simulink model "s3_22a"  (Simulink 6.6)
settings: Solver=FixedStepDiscrete  SolverMode=SingleTasking  StartTime=0.0  StopTime=t_d  FixedStep=Tc  MaxStep=Tc  RelTol=1e-6  AbsTol=1e-6
values from neighbouring files (symbols this model uses):
  a = [0.5; 0.5]    [i3_22.m]
  K = diag([500,500,500,100])    [i3_22.m]
  q_i = zeros(1,4)    [i3_22.m]
  Tc = 0.001    [i3_22.m]
  Ts = Tc    (= 0.001)    [i3_22.m]
undefined symbols (not defined in the file or in its folder): DiscIntNeverNeededParam
settings Model: Creator=luigivillani  LastModifiedBy=luigivillani  ExtModeAutoUpdateStatusClock=off
settings DataIOCC: LimitDataPoints=off  SaveOutput=off  SaveTime=off
settings OptimizationCC: BlockReduction=off  BooleanDataType=off
settings DebuggingCC: SignalResolutionControl=TryResolveAllWithWarning  SolverPrmCheckMsg=none  MultiTaskDSMMsg=warning  MultiTaskCondExecSysMsg=none  StrictBusMsg=None
settings HardwareCC: TargetUnknown=on
settings RTWCC: IncludeERTFirstTime=on

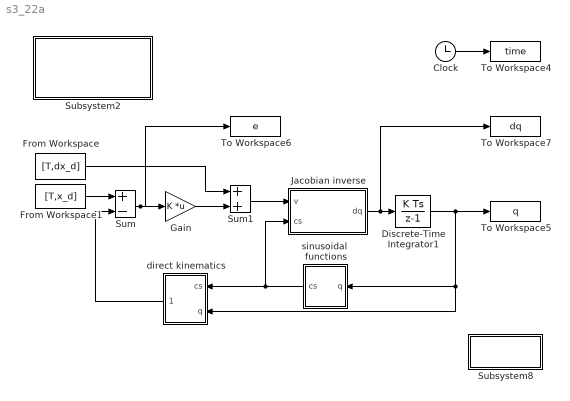
== system s3_22a ==
  Clock : Clock
  Discrete-Time Integrator1 : DiscreteIntegrator  InitialCondition=q_i  SampleTime=Tc  ICPrevOutput=DiscIntNeverNeededParam  ICPrevScaledInput=DiscIntNeverNeededParam
  From Workspace : FromWorkspace  VariableName=[T,dx_d]  SampleTime=Tc
  From Workspace1 : FromWorkspace  VariableName=[T,x_d]  SampleTime=Tc
  Gain : Gain  Gain=K  Multiplication=Matrix(K*u)  SampleTime=Tc
      mask Display: disp('K')
  Jacobian inverse : Subsystem
      mask Display: disp('inv(J_a(q))dx')
  Subsystem2 : Subsystem
      settings: OpenFcn=clear all;i3_22;
      mask Display: disp('variables\n initialization')
  Subsystem8 : Subsystem  Orientation=left
      settings: OpenFcn=p3_22a;
      mask Display: disp('plot')
  Sum : Sum  Inputs=+-  SaturateOnIntegerOverflow=on  InputSameDT=on
  Sum1 : Sum  SaturateOnIntegerOverflow=on  InputSameDT=on
  To Workspace4 : ToWorkspace  VariableName=time  SampleTime=Ts  SaveFormat=Array
      settings: MaxDataPoints=2501
  To Workspace5 : ToWorkspace  VariableName=q  SampleTime=Ts  SaveFormat=Array
      settings: MaxDataPoints=2501
  To Workspace6 : ToWorkspace  VariableName=e  SampleTime=Ts  SaveFormat=Array
      settings: MaxDataPoints=2501
  To Workspace7 : ToWorkspace  VariableName=dq  SampleTime=Ts  SaveFormat=Array
      settings: MaxDataPoints=2501
  direct kinematics : Subsystem  Orientation=left
      mask Display: disp('k(q)')
  sinusoidal  functions : Subsystem  Orientation=left
      mask Display: disp('cs(q)')
  wires:
  From Workspace1/1 -> Sum/1
  Clock/1 -> To Workspace4/1
  Gain/1 -> Sum1/2
  direct kinematics/1((x,y,z,phi)) -> Sum/2
  sinusoidal  functions/1(cs) -> direct kinematics/1(cs), Jacobian inverse/2(cs)
  Sum1/1 -> Jacobian inverse/1(v)
  Sum/1 -> To Workspace6/1, Gain/1
  From Workspace/1 -> Sum1/1
  Jacobian inverse/1(dq) -> To Workspace7/1, Discrete-Time Integrator1/1
  Discrete-Time Integrator1/1 -> To Workspace5/1, direct kinematics/2(q), sinusoidal  functions/1(q)

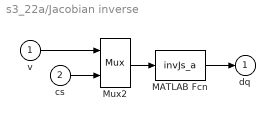
== system s3_22a/Jacobian inverse ==
  v : Inport
  cs : Inport  Port=2
  MATLAB Fcn : MATLABFcn  MATLABFcn=invJs_a  OutputDimensions=4
      mask Display: disp('invJ_a')
  Mux2 : Mux  Inputs=[4,4]
  dq : Outport  InitialOutput=0
  wires:
  cs/1 -> Mux2/2
  MATLAB Fcn/1 -> dq/1
  v/1 -> Mux2/1
  Mux2/1 -> MATLAB Fcn/1

== system s3_22a/Subsystem2 ==
  note: start

== system s3_22a/Subsystem8 ==
  note: start

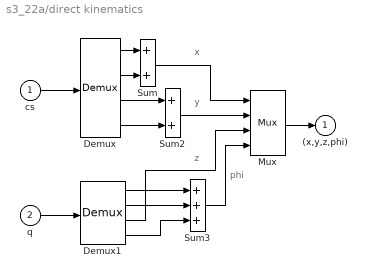
== system s3_22a/direct kinematics ==
  note: y
  note: x
  note: z
  note: phi
  cs : Inport
  q : Inport  Port=2
  Demux : Demux
  Demux1 : Demux
  Mux : Mux
  Sum : Sum  SaturateOnIntegerOverflow=on  InputSameDT=on
  Sum2 : Sum  SaturateOnIntegerOverflow=on  InputSameDT=on
  Sum3 : Sum  Inputs=+++  SaturateOnIntegerOverflow=on  InputSameDT=on
  (x,y,z,phi) : Outport  InitialOutput=0
  wires:
  Sum2/1 -> Mux/2
  q/1 -> Demux1/1
  Demux/2 -> Sum/2
  Mux/1 -> (x,y,z,phi)/1
  Sum/1 -> Mux/1
  Demux/1 -> Sum/1
  cs/1 -> Demux/1
  Demux/3 -> Sum2/1
  Demux/4 -> Sum2/2
  Demux1/2 -> Sum3/2
  Demux1/1 -> Sum3/1
  Demux1/4 -> Sum3/3
  Demux1/3 -> Mux/3
  Sum3/1 -> Mux/4

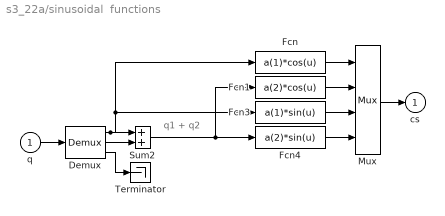
== system s3_22a/sinusoidal  functions ==
  note: q1 + q2
  q : Inport
  Demux : Demux  Outputs=[1,1,2]
  Fcn : Fcn  Expr=a(1)*cos(u)
  Fcn1 : Fcn  Expr=a(2)*cos(u)
  Fcn3 : Fcn  Expr=a(1)*sin(u)
  Fcn4 : Fcn  Expr=a(2)*sin(u)
  Mux : Mux
  Sum2 : Sum  SaturateOnIntegerOverflow=on  InputSameDT=on
  Terminator : Terminator
  cs : Outport  InitialOutput=0
  wires:
  q/1 -> Demux/1
  Demux/2 -> Sum2/2
  Mux/1 -> cs/1
  Fcn1/1 -> Mux/2
  Fcn/1 -> Mux/1
  Fcn3/1 -> Mux/3
  Fcn4/1 -> Mux/4
  Sum2/1 -> Fcn1/1, Fcn4/1
  Demux/1 -> Sum2/1, Fcn3/1, Fcn/1
  Demux/3 -> Terminator/1
